simulink model "Test1"  (R2022b)
settings: Solver=FixedStepAuto  StartTime=0.0  StopTime=100  FixedStep=1  RelTol=1e-3
undefined symbols (not defined in the file): sigbuilder_block, stamp
libraries: ros2lib x13, robotcorelib x1, robotmaniplib x1
settings Model: Creator=cosmin  LastModifiedBy=cosmin

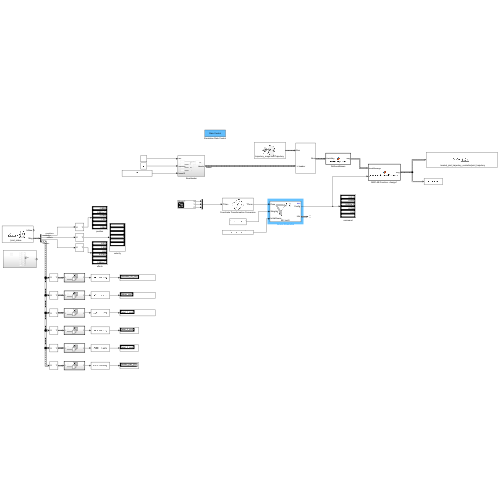
[thumbnail: Simulink's stored preview of the top-level diagram]
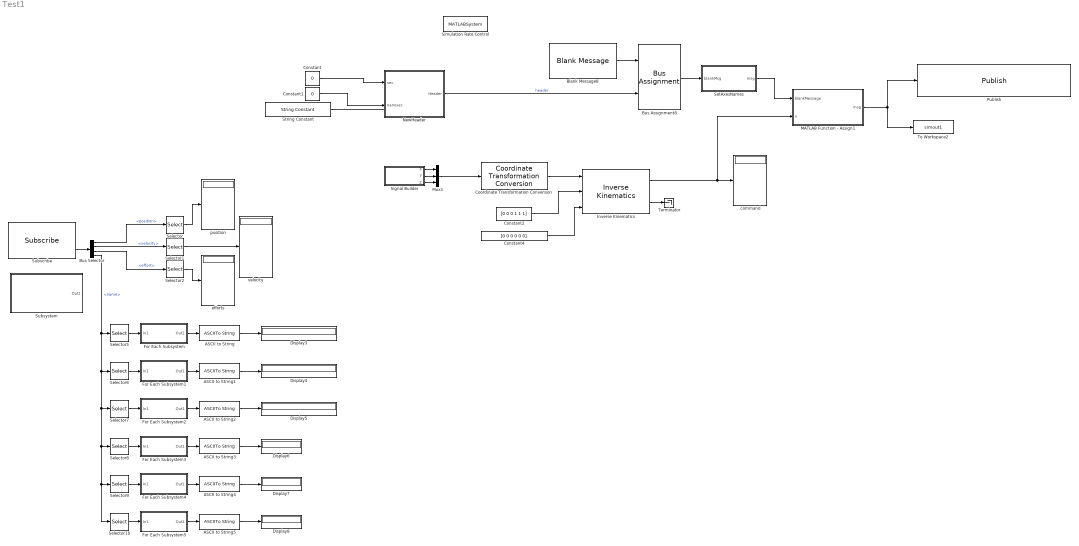
== system Test1 ==
  ASCII to String{,1..5} (6 alike) : ASCIIToString
  Blank Message8 : ros2lib/Blank Message  messageClass=Message  entityType=trajectory_msgs/JointTrajectory  messageType=trajectory_msgs/JointTrajectory  SampleTime=inf
      settings: LibrarySourceBlock=roslib/ROS 2/Blank Message
  Bus Assignment8 : BusAssignment  AssignedSignals=header
  Bus Selector : BusSelector  OutputSignals=position,velocity,effort,name
  Constant : Constant  Value=0  OutDataTypeStr=int32
  Constant1 : Constant  Value=0  OutDataTypeStr=uint32
  Constant2 : Constant  Value=[0 0 0 1 1 1]
  Constant4 : Constant  Value=[0 0 0 0 0 0]
  Coordinate Transformation Conversion : robotcorelib/Coordinate Transformation Conversion  InputRepresentation=Translation Vector  InputEulerSequence=ZYX  ShowTrVecInputPort=on  OutputRepresentation=Homogeneous Transformation  OutputEulerSequence=ZYX  ShowTrVecOutputPort=on  SimulateUsing=Interpreted execution
  Display{3..8} (6 alike) : Display
  For Each Subsystem : Subsystem  TreatAsAtomicUnit=on
  For Each Subsystem1 : Subsystem  TreatAsAtomicUnit=on
  For Each Subsystem2 : Subsystem  TreatAsAtomicUnit=on
  For Each Subsystem3 : Subsystem  TreatAsAtomicUnit=on
  For Each Subsystem4 : Subsystem  TreatAsAtomicUnit=on
  For Each Subsystem5 : Subsystem  TreatAsAtomicUnit=on
  Inverse Kinematics : robotmaniplib/Inverse Kinematics  RigidBodyTree=ans  EndEffector=tool0  ShowInfo=on  SolverName=BFGS Gradient Projection  EnforceJointLimits=on  MaxIterations=1500  MaxTime=10  GradientTolerance=1e-7  SolutionTolerance=1e-6  StepTolerance=1e-14  ErrorChangeTolerance=1e-12  UseErrorDamping=on  DampingBias=0.0025  SimulateUsing=Interpreted execution
  MATLAB Function - Assign1 : MATLAB Function  TreatAsAtomicUnit=on
  Mux1 : Mux  Inputs=3
  NewHeader : Subsystem
  Publish : ros2lib/Publish  topicSource=Select from ROS network  topic=/scaled_joint_trajectory_controller/joint_trajectory  messageType=trajectory_msgs/JointTrajectory  QOSHistory=Keep last  QOSDepth=1  QOSReliability=Reliable  QOSDurability=Volatile
      settings: LibrarySourceBlock=roslib/ROS 2/Publish
  Selector : Selector  InputPortWidth=128  IndexOptions=Index vector (dialog)  Indices=[1 2 3 4 5 6]  OutputSizes=1
  Selector1 : Selector  InputPortWidth=128  IndexOptions=Index vector (dialog)  Indices=[1 2 3 4 5 6]  OutputSizes=1
  Selector10 : Selector  InputPortWidth=16  IndexOptions=Index vector (dialog)  Indices=[6]  OutputSizes=1
  Selector2 : Selector  InputPortWidth=128  IndexOptions=Index vector (dialog)  Indices=[1 2 3 4 5 6]  OutputSizes=1
  Selector5 : Selector  InputPortWidth=16  IndexOptions=Index vector (dialog)  Indices=[1]  OutputSizes=1
  Selector6 : Selector  InputPortWidth=16  IndexOptions=Index vector (dialog)  Indices=[2]  OutputSizes=1
  Selector7 : Selector  InputPortWidth=16  IndexOptions=Index vector (dialog)  Indices=[3]  OutputSizes=1
  Selector8 : Selector  InputPortWidth=16  IndexOptions=Index vector (dialog)  Indices=[4]  OutputSizes=1
  Selector9 : Selector  InputPortWidth=16  IndexOptions=Index vector (dialog)  Indices=[5]  OutputSizes=1
  SetAxesNames : MATLAB Function  TreatAsAtomicUnit=on
  Signal Builder : Subsystem  Tag=STV Subsys  LoadFcn=sigbuilder_block('load');  StartFcn=sigbuilder_block('start');  StopFcn=sigbuilder_block('stop');  ClipboardFcn=sigbuilder_block('clipboard');  mask(Sigbuilder block){tuvar=[0:10]}
      mask help: Simulink:masks:SigbuilderBlock_MD
      mask init:
      | if ~strcmp(get_param(bdroot(gcbh),'SimulationStatus'),'stopped') tuvar = sigbuilder_block('maskInit'); end
      settings: CopyFcn=sigbuilder_block('copy');  DeleteFcn=sigbuilder_block('delete');  ModelCloseFcn=sigbuilder_block('modelClose');  PreSaveFcn=sigbuilder_block('preSave');  PauseFcn=sigbuilder_block('pause');  ContinueFcn=sigbuilder_block('continue');  NameChangeFcn=sigbuilder_block('namechange');  OpenFcn=sigbuilder_block('open',[437.6 92.4 579.4 493.8 ]);  CloseFcn=sigbuilder_block('close');
      mask Display: plot(0, 0, 100, 100,[2, 2, 32, 32, 2], [68, 8, 8, 68, 68],[32, 2], [38, 38], [32, 19, 2],[53, 60, 44], [32, 17, 17, 2],[16, 16, 31, 31]);txt = getActiveGroup(gcbh);text(2, 100, txt,'verticalAlignment', 'top');
  Simulation Rate Control : MATLABSystem  System=ExampleHelperSimulationRateControl  SampleTime=1
      mask Type: ExampleHelperSimulationRateControl
      mask Display: disp('Rate Control');
  String Constant : StringConstant  String="\"\""
  Subscribe : ros2lib/Subscribe  topicSource=Select from ROS network  topic=/joint_states  messageType=sensor_msgs/JointState  sampleTime=-1  QOSHistory=Keep last  QOSDepth=1  QOSReliability=Reliable  QOSDurability=Volatile
      settings: LibrarySourceBlock=roslib/ROS 2/Subscribe
  Subsystem : Subsystem
  Terminator : Terminator
  To Workspace2 : ToWorkspace  VariableName=simout1  SaveFormat=Timeseries  SampleTime=-1
  command : Display
  efforts : Display
  position : Display
  velocity : Display
  wires:
  String Constant/1 -> ?
  Constant1/1 -> NewHeader/2(nanosec)
  Constant/1 -> NewHeader/1(sec)
  NewHeader/1(Header) -> Bus Assignment8/2  "header"
  Blank Message8/1 -> Bus Assignment8/1
  Bus Assignment8/1 -> SetAxesNames/1(blankMsg)
  MATLAB Function - Assign1/1(msg) -> To Workspace2/1, Publish/1
  SetAxesNames/1(msg) -> MATLAB Function - Assign1/1(blankMessage)
  Subscribe/2 -> Bus Selector/1
  Bus Selector/1 -> Selector/1  "<position>"
  Selector/1 -> position/1
  Bus Selector/2 -> Selector1/1  "<velocity>"
  Bus Selector/3 -> Selector2/1  "<effort>"
  Selector1/1 -> velocity/1
  Selector2/1 -> efforts/1
  Bus Selector/4 -> Selector10/1, Selector9/1, Selector8/1, Selector7/1, Selector6/1, Selector5/1  "<name>"
  For Each Subsystem/1(Out1) -> ASCII to String/1
  Selector5/1 -> For Each Subsystem/1(In1)
  Selector6/1 -> For Each Subsystem1/1(In1)
  For Each Subsystem1/1(Out1) -> ASCII to String1/1
  ASCII to String/1 -> Display3/1
  ASCII to String1/1 -> Display4/1
  For Each Subsystem3/1(Out1) -> ASCII to String3/1
  Selector8/1 -> For Each Subsystem3/1(In1)
  Selector7/1 -> For Each Subsystem2/1(In1)
  For Each Subsystem2/1(Out1) -> ASCII to String2/1
  For Each Subsystem4/1(Out1) -> ASCII to String4/1
  Selector9/1 -> For Each Subsystem4/1(In1)
  Selector10/1 -> For Each Subsystem5/1(In1)
  For Each Subsystem5/1(Out1) -> ASCII to String5/1
  ASCII to String2/1 -> Display5/1
  ASCII to String3/1 -> Display6/1
  ASCII to String4/1 -> Display7/1
  ASCII to String5/1 -> Display8/1
  Constant4/1 -> Inverse Kinematics/3
  Signal Builder/1(X) -> Mux1/1
  Mux1/1 -> Coordinate Transformation Conversion/1
  Signal Builder/2(Y) -> Mux1/2
  Coordinate Transformation Conversion/1 -> Inverse Kinematics/1
  Signal Builder/3(Z) -> Mux1/3
  Inverse Kinematics/2 -> Terminator/1
  Constant2/1 -> Inverse Kinematics/2
  Inverse Kinematics/1 -> command/1, MATLAB Function - Assign1/2(u)

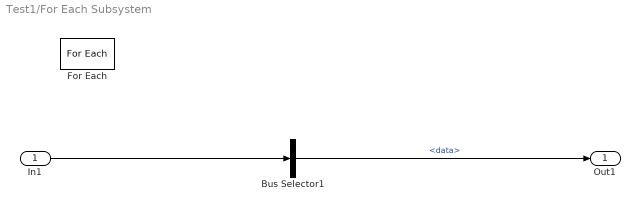
== system Test1/For Each Subsystem ==
  In1 : Inport  Partition=on  PartitionDimension=1  PartitionWidth=1  PartitionOffset=0
  Bus Selector1 : BusSelector  OutputSignals=data
  For Each : ForEach  DisableCoverage=on
  Out1 : Outport  ConcatenationDimension=1
  wires:
  In1/1 -> Bus Selector1/1
  Bus Selector1/1 -> Out1/1  "<data>"

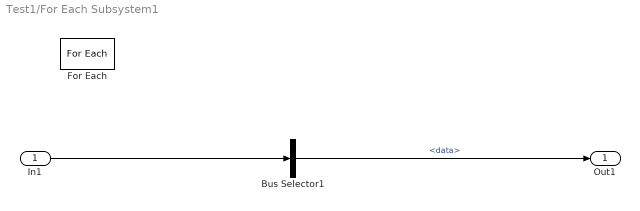
== system Test1/For Each Subsystem1 ==
  In1 : Inport  Partition=on  PartitionDimension=1  PartitionWidth=1  PartitionOffset=0
  Bus Selector1 : BusSelector  OutputSignals=data
  For Each : ForEach  DisableCoverage=on
  Out1 : Outport  ConcatenationDimension=1
  wires:
  Bus Selector1/1 -> Out1/1  "<data>"
  In1/1 -> Bus Selector1/1

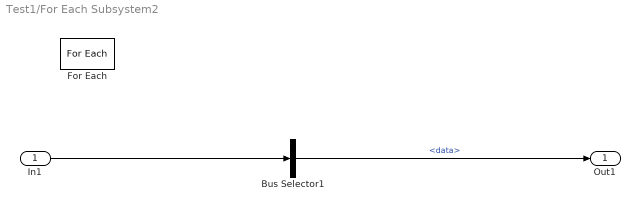
== system Test1/For Each Subsystem2 ==
  In1 : Inport  Partition=on  PartitionDimension=1  PartitionWidth=1  PartitionOffset=0
  Bus Selector1 : BusSelector  OutputSignals=data
  For Each : ForEach  DisableCoverage=on
  Out1 : Outport  ConcatenationDimension=1
  wires:
  Bus Selector1/1 -> Out1/1  "<data>"
  In1/1 -> Bus Selector1/1

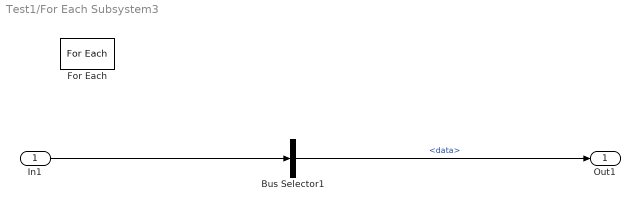
== system Test1/For Each Subsystem3 ==
  In1 : Inport  Partition=on  PartitionDimension=1  PartitionWidth=1  PartitionOffset=0
  Bus Selector1 : BusSelector  OutputSignals=data
  For Each : ForEach  DisableCoverage=on
  Out1 : Outport  ConcatenationDimension=1
  wires:
  In1/1 -> Bus Selector1/1
  Bus Selector1/1 -> Out1/1  "<data>"

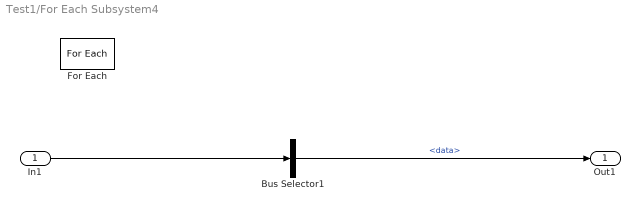
== system Test1/For Each Subsystem4 ==
  In1 : Inport  Partition=on  PartitionDimension=1  PartitionWidth=1  PartitionOffset=0
  Bus Selector1 : BusSelector  OutputSignals=data
  For Each : ForEach  DisableCoverage=on
  Out1 : Outport  ConcatenationDimension=1
  wires:
  In1/1 -> Bus Selector1/1
  Bus Selector1/1 -> Out1/1  "<data>"

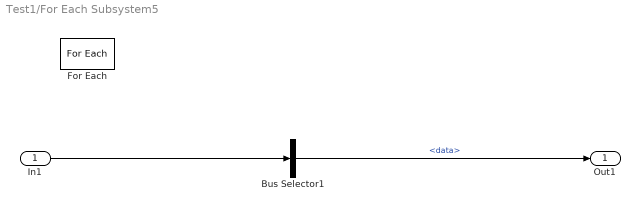
== system Test1/For Each Subsystem5 ==
  In1 : Inport  Partition=on  PartitionDimension=1  PartitionWidth=1  PartitionOffset=0
  Bus Selector1 : BusSelector  OutputSignals=data
  For Each : ForEach  DisableCoverage=on
  Out1 : Outport  ConcatenationDimension=1
  wires:
  Bus Selector1/1 -> Out1/1  "<data>"
  In1/1 -> Bus Selector1/1

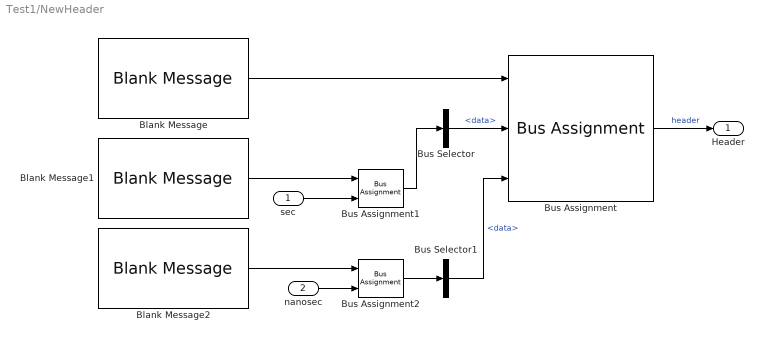
== system Test1/NewHeader ==
  sec : Inport  OutDataTypeStr=int32
  nanosec : Inport  Port=2  OutDataTypeStr=uint32
  Blank Message : ros2lib/Blank Message  messageClass=Message  entityType=std_msgs/Header  messageType=std_msgs/Header  SampleTime=inf
      settings: LibrarySourceBlock=roslib/ROS 2/Blank Message
  Blank Message1 : ros2lib/Blank Message  messageClass=Message  entityType=std_msgs/Int32  messageType=std_msgs/Int32  SampleTime=inf
      settings: LibrarySourceBlock=roslib/ROS 2/Blank Message
  Blank Message2 : ros2lib/Blank Message  messageClass=Message  entityType=std_msgs/UInt32  messageType=std_msgs/UInt32  SampleTime=inf
      settings: LibrarySourceBlock=roslib/ROS 2/Blank Message
  Bus Assignment : BusAssignment  AssignedSignals=stamp.sec,stamp.nanosec
  Bus Assignment1 : BusAssignment  AssignedSignals=data
  Bus Assignment2 : BusAssignment  AssignedSignals=data
  Bus Selector : BusSelector  OutputSignals=data
  Bus Selector1 : BusSelector  OutputSignals=data
  Header : Outport
  wires:
  Bus Assignment/1 -> Header/1  "header"
  nanosec/1 -> Bus Assignment2/2
  Blank Message1/1 -> Bus Assignment1/1
  Bus Assignment1/1 -> Bus Selector/1
  Blank Message/1 -> Bus Assignment/1
  sec/1 -> Bus Assignment1/2
  Blank Message2/1 -> Bus Assignment2/1
  Bus Selector/1 -> Bus Assignment/2  "<data>"
  Bus Assignment2/1 -> Bus Selector1/1
  Bus Selector1/1 -> Bus Assignment/3  "<data>"

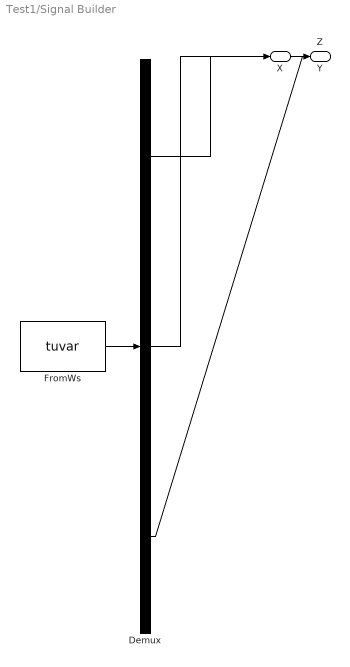
== system Test1/Signal Builder ==
  Demux : Demux  Tag=STV Demux  Outputs=3
      settings: DisplayOption=none
  FromWs : FromWorkspace  Tag=STV FromWs  VariableName=tuvar
      SigBuilderData=|
      | common.afterFinalStr = 'Extrapolate'
      | common.sampleTime = 0
      | dataSet.timeRange = [0 10]
      | dataSet.name = 'Group 1'
      | sbobj.Groups.Name = 'Group 1'
      | sbobj.Groups.Signals(1).Name = 'X'
      | sbobj.Groups.Signals(1).XData = [0 1 2 3 4 5 10]
      | sbobj.Groups.Signals(1).YData = [0.39 0.31 0.25 0.22 0.235 0.306 0.395]
      | sbobj.Groups.Signals(2).Name = 'Y'
      | sbobj.Groups.Signals(2).XData = [0 1 2 3 4 10]
      | sbobj.Groups.Signals(2).YData = [1 1 1 1 1 1]
      | sbobj.Groups.Signals(3).Name = 'Z'
      | sbobj.Groups.Signals(3).XData = [0 1 2 3 4 10]
      | sbobj.Groups.Signals(3).YData = [2 2 2 2 2 2]
  X : Outport  Tag=STV Outport
  Y : Outport  Tag=STV Outport  Port=2
  Z : Outport  Tag=STV Outport  Port=3
  wires:
  FromWs/1 -> Demux/1
  Demux/1 -> X/1
  Demux/2 -> Y/1
  Demux/3 -> Z/1

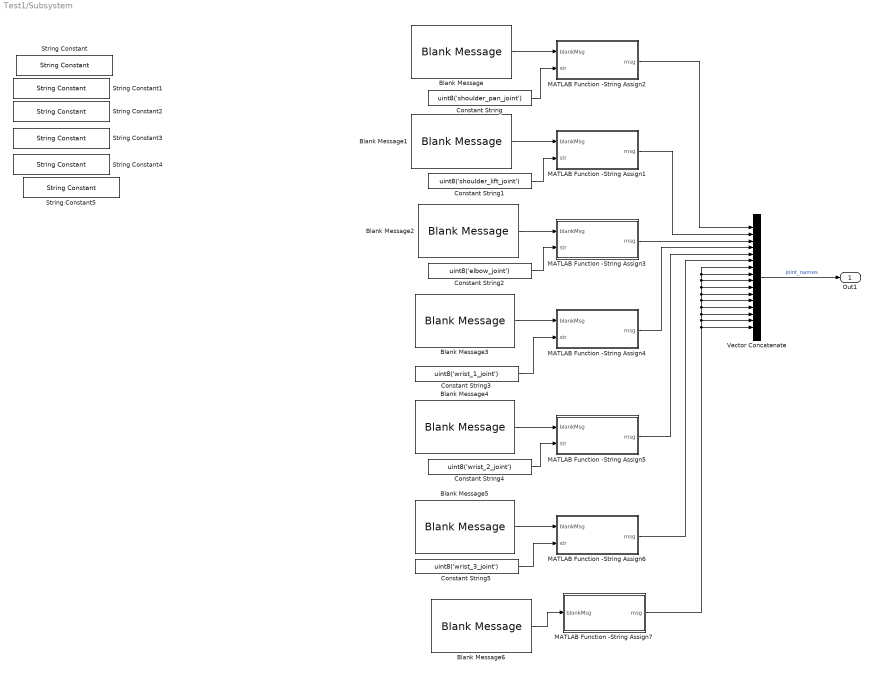
== system Test1/Subsystem ==
  Blank Message{,1..6} (7 alike) : ros2lib/Blank Message  messageClass=Message  entityType=std_msgs/String  messageType=std_msgs/String  SampleTime=inf
      settings: LibrarySourceBlock=roslib/ROS 2/Blank Message
  Constant String : Constant  Value=uint8('shoulder_pan_joint')
  Constant String1 : Constant  Value=uint8('shoulder_lift_joint')
  Constant String2 : Constant  Value=uint8('elbow_joint')
  Constant String3 : Constant  Value=uint8('wrist_1_joint')
  Constant String4 : Constant  Value=uint8('wrist_2_joint')
  Constant String5 : Constant  Value=uint8('wrist_3_joint')
  MATLAB Function -String Assign1 : MATLAB Function  TreatAsAtomicUnit=on
  MATLAB Function -String Assign2 : MATLAB Function  TreatAsAtomicUnit=on
  MATLAB Function -String Assign3 : MATLAB Function  TreatAsAtomicUnit=on
  MATLAB Function -String Assign4 : MATLAB Function  TreatAsAtomicUnit=on
  MATLAB Function -String Assign5 : MATLAB Function  TreatAsAtomicUnit=on
  MATLAB Function -String Assign6 : MATLAB Function  TreatAsAtomicUnit=on
  MATLAB Function -String Assign7 : MATLAB Function  TreatAsAtomicUnit=on
  String Constant : StringConstant  String="\"shoulder_pan_joint\""
  String Constant1 : StringConstant  String="\"shoulder_lift_joint\""
  String Constant2 : StringConstant  String="\"elbow_joint\""
  String Constant3 : StringConstant  String="\"wrist_1_joint\""
  String Constant4 : StringConstant  String="\"wrist_2_joint\""
  String Constant5 : StringConstant  String="\"wrist_3_joint\""
  Vector Concatenate : Concatenate  NumInputs=16
  Out1 : Outport
  wires:
  Vector Concatenate/1 -> Out1/1  "joint_names"
  Constant String/1 -> MATLAB Function -String Assign2/2(str)
  Constant String1/1 -> MATLAB Function -String Assign1/2(str)
  Constant String2/1 -> MATLAB Function -String Assign3/2(str)
  Constant String3/1 -> MATLAB Function -String Assign4/2(str)
  Constant String5/1 -> MATLAB Function -String Assign6/2(str)
  Blank Message5/1 -> MATLAB Function -String Assign6/1(blankMsg)
  Constant String4/1 -> MATLAB Function -String Assign5/2(str)
  Blank Message4/1 -> MATLAB Function -String Assign5/1(blankMsg)
  Blank Message3/1 -> MATLAB Function -String Assign4/1(blankMsg)
  Blank Message2/1 -> MATLAB Function -String Assign3/1(blankMsg)
  Blank Message1/1 -> MATLAB Function -String Assign1/1(blankMsg)
  Blank Message/1 -> MATLAB Function -String Assign2/1(blankMsg)
  MATLAB Function -String Assign2/1(msg) -> Vector Concatenate/1
  MATLAB Function -String Assign1/1(msg) -> Vector Concatenate/2
  MATLAB Function -String Assign3/1(msg) -> Vector Concatenate/3
  MATLAB Function -String Assign4/1(msg) -> Vector Concatenate/4
  MATLAB Function -String Assign5/1(msg) -> Vector Concatenate/5
  MATLAB Function -String Assign6/1(msg) -> Vector Concatenate/6
  MATLAB Function -String Assign7/1(msg) -> Vector Concatenate/16, Vector Concatenate/15, Vector Concatenate/14, Vector Concatenate/13, Vector Concatenate/12, Vector Concatenate/11, Vector Concatenate/10, Vector Concatenate/9, Vector Concatenate/8, Vector Concatenate/7
  Blank Message6/1 -> MATLAB Function -String Assign7/1(blankMsg)

== matlab function Test1/Subsystem/MATLAB Function -String Assign1 ==
  data: blankMsg input Bus: SL_Bus_std_msgs_String; msg output Bus: SL_Bus_std_msgs_String; str input
function msg = assignStringInput(blankMsg, str)
% assignStringInput - Assign a string in a ROS message to specified input string
%
% MSG = assignStringInput(blankMsg, STR) assigns the input string, STR, to
%  a string field in the ROS message, blankMsg, and outputs the updated
%  ROS message.
%
%  Inputs
%    blankMsg: A bus for a 'std_msgs/String' message. This is 
%        used to initialize the output.
%    str: An array of uint8 that will be assigned to the 'Data' field
%        in blankMsg. The entire array is assumed to be a valid sequence of
%        character ASCII values.
% 
%  Outputs:
%    msg: A bus for a 'std_msgs/String' message, with the 'Data'
%        field set to a string.

%   Copyright 2015 The MathWorks, Inc.
%#codegen

% Note: The datatype of 'msg' has been explicitly set to the appropriate 
% Simulink bus type ("Bus: SL_Bus_robotROSMessageUsageExample_std_msgs_String"). 
%
% If the model name is changed, the datatype needs to be changed as well:
%   1) Click "Edit Data" in the Editor toolstrip to open "Ports and Data Manager"
%   2) Select "msg". From the "Type" dropdown, select "--- Refresh data types ---"
%   3) Set datatype to "Bus: SL_Bus_<modelname>_std_msgs_String"
    
msg = blankMsg;

% msg (std_msgs/String) consists of
%           Data : array of type uint8
%   Data_SL_Info : struct with fields CurrentLength, ReceivedLength
strLength = length(str);
msg.data(1:strLength) = str;
msg.data_SL_Info.CurrentLength = uint32(strLength);

== matlab function Test1/Subsystem/MATLAB Function -String Assign3 ==
  data: blankMsg input Bus: SL_Bus_std_msgs_String; msg output Bus: SL_Bus_std_msgs_String; str input
function msg = assignStringInput(blankMsg, str)
% assignStringInput - Assign a string in a ROS message to specified input string
%
% MSG = assignStringInput(blankMsg, STR) assigns the input string, STR, to
%  a string field in the ROS message, blankMsg, and outputs the updated
%  ROS message.
%
%  Inputs
%    blankMsg: A bus for a 'std_msgs/String' message. This is 
%        used to initialize the output.
%    str: An array of uint8 that will be assigned to the 'Data' field
%        in blankMsg. The entire array is assumed to be a valid sequence of
%        character ASCII values.
% 
%  Outputs:
%    msg: A bus for a 'std_msgs/String' message, with the 'Data'
%        field set to a string.

%   Copyright 2015 The MathWorks, Inc.
%#codegen

% Note: The datatype of 'msg' has been explicitly set to the appropriate 
% Simulink bus type ("Bus: SL_Bus_robotROSMessageUsageExample_std_msgs_String"). 
%
% If the model name is changed, the datatype needs to be changed as well:
%   1) Click "Edit Data" in the Editor toolstrip to open "Ports and Data Manager"
%   2) Select "msg". From the "Type" dropdown, select "--- Refresh data types ---"
%   3) Set datatype to "Bus: SL_Bus_<modelname>_std_msgs_String"
    
msg = blankMsg;

% msg (std_msgs/String) consists of
%           Data : array of type uint8
%   Data_SL_Info : struct with fields CurrentLength, ReceivedLength
strLength = length(str);
msg.data(1:strLength) = str;
msg.data_SL_Info.CurrentLength = uint32(strLength);

== matlab function Test1/Subsystem/MATLAB Function -String Assign2 ==
  data: blankMsg input Bus: SL_Bus_std_msgs_String; msg output Bus: SL_Bus_std_msgs_String; str input
function msg = assignStringInput(blankMsg, str)
% assignStringInput - Assign a string in a ROS message to specified input string
%
% MSG = assignStringInput(blankMsg, STR) assigns the input string, STR, to
%  a string field in the ROS message, blankMsg, and outputs the updated
%  ROS message.
%
%  Inputs
%    blankMsg: A bus for a 'std_msgs/String' message. This is 
%        used to initialize the output.
%    str: An array of uint8 that will be assigned to the 'Data' field
%        in blankMsg. The entire array is assumed to be a valid sequence of
%        character ASCII values.
% 
%  Outputs:
%    msg: A bus for a 'std_msgs/String' message, with the 'Data'
%        field set to a string.

%   Copyright 2015 The MathWorks, Inc.
%#codegen

% Note: The datatype of 'msg' has been explicitly set to the appropriate 
% Simulink bus type ("Bus: SL_Bus_robotROSMessageUsageExample_std_msgs_String"). 
%
% If the model name is changed, the datatype needs to be changed as well:
%   1) Click "Edit Data" in the Editor toolstrip to open "Ports and Data Manager"
%   2) Select "msg". From the "Type" dropdown, select "--- Refresh data types ---"
%   3) Set datatype to "Bus: SL_Bus_<modelname>_std_msgs_String"
    
msg = blankMsg;

% msg (std_msgs/String) consists of
%           Data : array of type uint8
%   Data_SL_Info : struct with fields CurrentLength, ReceivedLength
strLength = length(str);
msg.data(1:strLength) = str;
msg.data_SL_Info.CurrentLength = uint32(strLength);

== matlab function Test1/Subsystem/MATLAB Function -String Assign4 ==
  data: blankMsg input Bus: SL_Bus_std_msgs_String; msg output Bus: SL_Bus_std_msgs_String; str input
function msg = assignStringInput(blankMsg, str)
% assignStringInput - Assign a string in a ROS message to specified input string
%
% MSG = assignStringInput(blankMsg, STR) assigns the input string, STR, to
%  a string field in the ROS message, blankMsg, and outputs the updated
%  ROS message.
%
%  Inputs
%    blankMsg: A bus for a 'std_msgs/String' message. This is 
%        used to initialize the output.
%    str: An array of uint8 that will be assigned to the 'Data' field
%        in blankMsg. The entire array is assumed to be a valid sequence of
%        character ASCII values.
% 
%  Outputs:
%    msg: A bus for a 'std_msgs/String' message, with the 'Data'
%        field set to a string.

%   Copyright 2015 The MathWorks, Inc.
%#codegen

% Note: The datatype of 'msg' has been explicitly set to the appropriate 
% Simulink bus type ("Bus: SL_Bus_robotROSMessageUsageExample_std_msgs_String"). 
%
% If the model name is changed, the datatype needs to be changed as well:
%   1) Click "Edit Data" in the Editor toolstrip to open "Ports and Data Manager"
%   2) Select "msg". From the "Type" dropdown, select "--- Refresh data types ---"
%   3) Set datatype to "Bus: SL_Bus_<modelname>_std_msgs_String"
    
msg = blankMsg;

% msg (std_msgs/String) consists of
%           Data : array of type uint8
%   Data_SL_Info : struct with fields CurrentLength, ReceivedLength
strLength = length(str);
msg.data(1:strLength) = str;
msg.data_SL_Info.CurrentLength = uint32(strLength);

== matlab function Test1/Subsystem/MATLAB Function -String Assign5 ==
  data: blankMsg input Bus: SL_Bus_std_msgs_String; msg output Bus: SL_Bus_std_msgs_String; str input
function msg = assignStringInput(blankMsg, str)
% assignStringInput - Assign a string in a ROS message to specified input string
%
% MSG = assignStringInput(blankMsg, STR) assigns the input string, STR, to
%  a string field in the ROS message, blankMsg, and outputs the updated
%  ROS message.
%
%  Inputs
%    blankMsg: A bus for a 'std_msgs/String' message. This is 
%        used to initialize the output.
%    str: An array of uint8 that will be assigned to the 'Data' field
%        in blankMsg. The entire array is assumed to be a valid sequence of
%        character ASCII values.
% 
%  Outputs:
%    msg: A bus for a 'std_msgs/String' message, with the 'Data'
%        field set to a string.

%   Copyright 2015 The MathWorks, Inc.
%#codegen

% Note: The datatype of 'msg' has been explicitly set to the appropriate 
% Simulink bus type ("Bus: SL_Bus_robotROSMessageUsageExample_std_msgs_String"). 
%
% If the model name is changed, the datatype needs to be changed as well:
%   1) Click "Edit Data" in the Editor toolstrip to open "Ports and Data Manager"
%   2) Select "msg". From the "Type" dropdown, select "--- Refresh data types ---"
%   3) Set datatype to "Bus: SL_Bus_<modelname>_std_msgs_String"
    
msg = blankMsg;

% msg (std_msgs/String) consists of
%           Data : array of type uint8
%   Data_SL_Info : struct with fields CurrentLength, ReceivedLength
strLength = length(str);
msg.data(1:strLength) = str;
msg.data_SL_Info.CurrentLength = uint32(strLength);

== matlab function Test1/Subsystem/MATLAB Function -String Assign6 ==
  data: blankMsg input Bus: SL_Bus_std_msgs_String; msg output Bus: SL_Bus_std_msgs_String; str input
function msg = assignStringInput(blankMsg, str)
% assignStringInput - Assign a string in a ROS message to specified input string
%
% MSG = assignStringInput(blankMsg, STR) assigns the input string, STR, to
%  a string field in the ROS message, blankMsg, and outputs the updated
%  ROS message.
%
%  Inputs
%    blankMsg: A bus for a 'std_msgs/String' message. This is 
%        used to initialize the output.
%    str: An array of uint8 that will be assigned to the 'Data' field
%        in blankMsg. The entire array is assumed to be a valid sequence of
%        character ASCII values.
% 
%  Outputs:
%    msg: A bus for a 'std_msgs/String' message, with the 'Data'
%        field set to a string.

%   Copyright 2015 The MathWorks, Inc.
%#codegen

% Note: The datatype of 'msg' has been explicitly set to the appropriate 
% Simulink bus type ("Bus: SL_Bus_robotROSMessageUsageExample_std_msgs_String"). 
%
% If the model name is changed, the datatype needs to be changed as well:
%   1) Click "Edit Data" in the Editor toolstrip to open "Ports and Data Manager"
%   2) Select "msg". From the "Type" dropdown, select "--- Refresh data types ---"
%   3) Set datatype to "Bus: SL_Bus_<modelname>_std_msgs_String"
    
msg = blankMsg;

% msg (std_msgs/String) consists of
%           Data : array of type uint8
%   Data_SL_Info : struct with fields CurrentLength, ReceivedLength
strLength = length(str);
msg.data(1:strLength) = str;
msg.data_SL_Info.CurrentLength = uint32(strLength);

== matlab function Test1/Subsystem/MATLAB Function -String Assign7 ==
  data: blankMsg input Bus: SL_Bus_std_msgs_String; msg output Bus: SL_Bus_std_msgs_String
function msg = assignString(blankMsg)
% assignString - Assign a string in a ROS message
%
% MSG = assignString(blankMsg) assigns a known string value to a 
%  string field in a ROS message, and outputs the updated ROS message.
%
%  blankMsg (input): A bus for a 'std_msgs/String' message. This is 
%      used to initialize the output. 
%  msg (output): A bus for a 'std_msgs/String' message, with the Data 
%      field set to a string.

%   Copyright 2015 The MathWorks, Inc.
%#codegen

% Note: The datatype of 'msg' has been explicitly set to the appropriate 
% Simulink bus type ("Bus: SL_Bus_robotROSMessageUsageExample_std_msgs_String"). 
%
% If the model name is changed, the datatype needs to be changed as well:
%   1) Click "Edit Data" in the Editor toolstrip to open "Ports and Data Manager"
%   2) Select "msg". From the "Type" dropdown, select "--- Refresh data types ---"
%   3) Set datatype to "Bus: SL_Bus_<modelname>_std_msgs_String"
    
stringToAssign = 'information';
msg = blankMsg;

% msg (std_msgs/String) consists of
%           Data : array of type uint8
%   Data_SL_Info : struct with fields CurrentLength, ReceivedLength
strLength = length(stringToAssign);
msg.data(1:strLength) = uint8(stringToAssign);
msg.data_SL_Info.CurrentLength = uint32(strLength);

== matlab function Test1/SetAxesNames ==
  data: blankMsg input Bus: SL_Bus_trajectory_msgs_JointTrajectory; msg output Bus: SL_Bus_trajectory_msgs_JointTrajectory
function msg = stringArrayAssign(blankMsg)
% stringArrayAssign - Assign a string array in a ROS message
%
%  blankMsg (input): A bus for a 'sensor_msgs/JointState' message. This is 
%      used to initialize the output.
%  msg (output): A bus for a 'sensor_msgs/JointState' message message, with 
%      Name field set to a string array.
%
%   Copyright 2015 The MathWorks, Inc.

%#codegen

% Note: The datatype of 'msg' has been explicitly set to the appropriate 
% Simulink bus type ("SL_Bus_robotROSMessageUsageExample_sensor_msgs_JointState"). 
%
% If the model name is changed, the datatype needs to be changed as well:
%   1) Click "Edit Data" in the Editor toolstrip to open "Ports and Data Manager"
%   2) Select "msg". From the "Type" dropdown, select "--- Refresh data types ---"
%   3) Set datatype to "Bus: SL_Bus_<modelname>_sensor_msgs_JointState"

strArrayToAssign = {'shoulder_pan_joint'; 'shoulder_lift_joint'; 'elbow_joint'; 'wrist_1_joint';'wrist_2_joint';'wrist_3_joint'};
msg = blankMsg;

% Set the number of strings in the string array.
% msg (sensor_msgs/JointState) includes the following fields
%           Name : array of std_msgs/String (string array)
%   Name_SL_Info : struct with fields CurrentLength, ReceivedLength
numStringsInArray = length(strArrayToAssign);
msg.joint_names_SL_Info.CurrentLength = uint32(numStringsInArray);

% Set the individual strings in the array
for idx=1:numStringsInArray
    str = strArrayToAssign{idx};
    strLength = length(str);
    msg.joint_names(idx).data(1:strLength) = uint8(str);
    msg.joint_names(idx).data_SL_Info.CurrentLength = uint32(strLength);
end

== matlab function Test1/MATLAB Function - Assign1 ==
  data: blankMessage input Bus: SL_Bus_trajectory_msgs_JointTrajectory; u input; msg output Bus: SL_Bus_trajectory_msgs_JointTrajectory
function msg = assignNestedArrayMessages(blankMessage,u)
%#codegen

% To set datatype of MSG output:
%  1. Create buses for this model: robotics.ros.createSimulinkBus(gcs)
%  1. Click "Edit Data" in  Toolstrip to open "Ports and Data Manager"
%  2. Select MSG and set datatype to "Bus: SL_Bus_<modelname>_<messageType>"
% See: 
% http://www.mathworks.com/help/simulink/ug/create-structures-in-matlab-function-blocks.html

% blankMessage (geometry_msgs/PoseArray) consists of
%          Header: [1x1 Header]
%           Poses: variable-length array of geometry_msgs/Pose
%   Poses_SL_Info: struct with fields CurrentLength, ReceivedLength
%
% Poses is an array of "geometry_msgs/Pose", which consists of
%        Position: [1x1 Point]
%     Orientation: [1x1 Quaternion]
%
% Position is "geometry_msgs/Point", which consists of
%               X: 0
%               Y: 0
%               Z: 0
%
% Orientation is "geometry_msgs/Quaternion", which consists of
%               X: 0
%               Y: 0
%               Z: 0
%               W: 0

% Set the Poses array to have size 2, and modify the first two Pose
% elements

blankMessage.points_SL_Info.CurrentLength = uint32(1);
blankMessage.points(1).positions_SL_Info.CurrentLength=uint32(6);
blankMessage.points(1).positions(1) = u(1);
blankMessage.points(1).positions(2) = u(2);
blankMessage.points(1).positions(3) = u(3);
blankMessage.points(1).positions(4) = u(4);
blankMessage.points(1).positions(5) = u(5);
blankMessage.points(1).positions(6) = u(6);

%blankMessage.layout.Dim(1).Size = uint32(size(u,1));
%blankMessage.layout.Dim(2).Size = uint32(size(u,2));
%blankMessage.layout.Dim(1).Stride = uint32(prod(size(u)));
%blankMessage.layout.Dim(2).Stride = uint32(prod(size(u,2)));

msg = blankMessage;
